simulink model "AB_Final_of_MPC_Bandwidth_Result_UnbalancedNew"  (R2022b)
settings: Solver=FixedStepDiscrete  StartTime=0.0  StopTime=Inf  FixedStep=100e-6  RelTol=1e-3  EnableMultiTasking=on
undefined symbols (not defined in the file): C28x, CPU1, CPU2, CurrentBypassValue, DiscIntNeverNeededParam, Down, GPTRIP1SEL, TZ1, Up
libraries: c2802xlib x20, simulink x17, dspstat3 x13, eeGeneralControl x10, c2837xDlib x5, c280xlib x5, PID_Lib x4, c2000lib x1, spsAlphaBetaZerotoabcLib x1
(part 2 of 10)

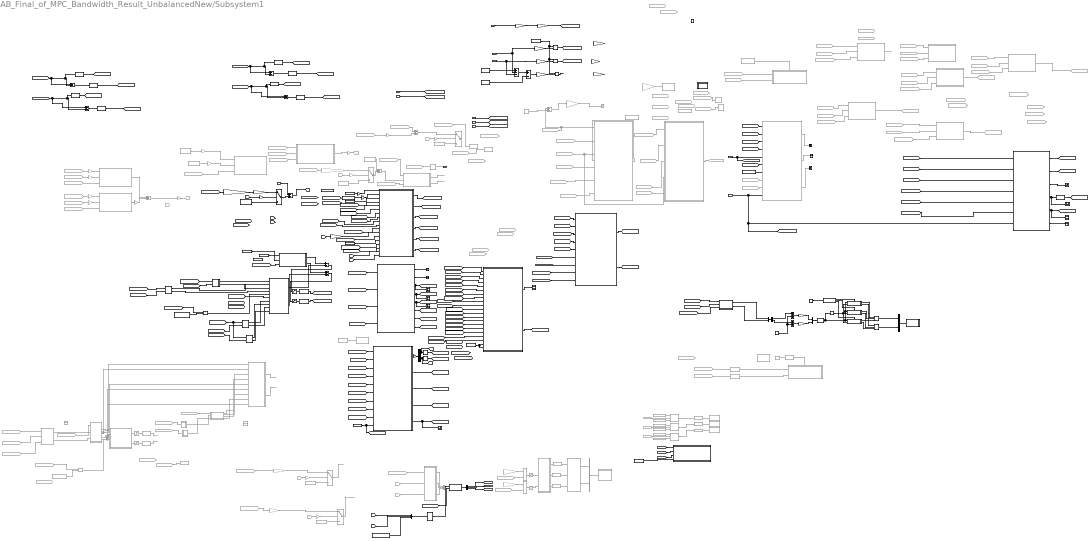
== system AB_Final_of_MPC_Bandwidth_Result_UnbalancedNew/Subsystem1 ==
  MPCC_f32GridCurrentA : Inport
  MPCC_f32GridCurrentB : Inport  Port=2
  PI_f32GridVoltageA : Inport  Port=3
  PI_f32GridVoltageB : Inport  Port=4
  PI_f32GridVoltageC : Inport  Port=5
  PI_f32DGridCurrentReference : Inport  Port=6
  PI_f32AngularFrequency : Inport  Port=7
  PI_f32ElectricalAngle : Inport  Port=8
  PI_f32DCLinkVoltage : Inport  Port=9
  PI_f32DCLinkVoltageref : Inport  Port=10
  MPCC_f32GridCurrentC : Inport  Port=11
  function : TriggerPort  TriggerType=function-call  VariantControl=(inherit)
  ABCtoAlphaBeta : Subsystem  Commented=on
  ABCtoD : Subsystem  Commented=on
  ABCtoD1Pos : Subsystem  Commented=on
  ABCtoD1Pos1 : Subsystem  Commented=on
  ABCtoD1Pos2 : Subsystem  Commented=on
  ABCtoD2 : Subsystem  Commented=on
  ABCtoD2Neg : Subsystem  Commented=on
  ABCtoD2Neg1 : Subsystem  Commented=on
  ABCtoD3 : Subsystem  Commented=on
  ABCtoDQO : Subsystem
  ABCtoQ : Subsystem  Commented=on
  ABCtoQPos1 : Subsystem  Commented=on
  Add1 : Sum  Inputs=+--
  Add{3,5,11,13..14} (5 alike) : Sum
  Add{4,6..7,12} (4 alike) : Sum  Commented=on
  Add{2,8..9,15..16} (5 alike) : Sum  Inputs=+-
  Alpha-Beta-Zero to abc : spsAlphaBetaZerotoabcLib/Alpha-Beta-Zero to abc
      settings: LibrarySourceBlock=|
      | sps_lib/Control/Alpha-Beta-Zero
      | to abc
  AlphaBetaDutiesCalculation : Subsystem
  AlphaBetaVoltageReferenceCalculation : Subsystem  Commented=on
  AlphaBetaVoltageReferenceCalculation1 : Subsystem
  "Angle_Identification " : Subsystem  Commented=on
  Bus Creator1 : BusCreator  Inputs=2
  Bus Selector2 : BusSelector  OutputSignals=signal1,signal2
  Cast To Boolean : DataTypeConversion  Commented=on  OutDataTypeStr=boolean  SaturateOnIntegerOverflow=off  RndMeth=Floor
  Cast To Single{,1..3,9..10,13..16,21} (11 alike) : DataTypeConversion  Commented=on  OutDataTypeStr=single  SaturateOnIntegerOverflow=off  RndMeth=Floor
  Cast To Single{6..8,11..12,17..20,22..23} (11 alike) : DataTypeConversion  OutDataTypeStr=single  SaturateOnIntegerOverflow=off  RndMeth=Floor
  CodeGeneration1 : Subsystem  TreatAsAtomicUnit=on
  Constant : Constant  Value=single(18.355e-3)
  Constant{1,10..11,14,48,50} (6 alike) : Constant  Value=single(0)
  Constant12 : Constant  Commented=on  Value=uint32(4999)
  Constant13 : Constant  Commented=on  Value=uint32(0)
  Constant{9,15,35,52,54} (5 alike) : Constant  Commented=on  Value=single(0)
  Constant16 : Constant  Commented=on  Value=uint32(4999)
  Constant17 : Constant  Commented=on  Value=uint32(0)
  Constant18 : Constant  Value=single(300)
  Constant19 : Constant  Value=single(9.5e-3)
  Constant2 : Constant  Value=single(0.005)
  Constant20 : Constant  Value=single(0.34)
  Constant21 : Constant  Value=single(18.5825e-3)
  Constant22 : Constant  Value=single(100e-6)
  Constant23 : Constant  Commented=on  Value=single(300)
  Constant26 : Constant  Value=single(1/10000)
  Constant3 : Constant  Value=10  OutDataTypeStr=single
  Constant36 : Constant  Commented=on
  Constant37 : Constant  Commented=on  Value=boolean(1)
  Constant4 : Constant  Commented=on  Value=single(1)  VectorParams1D=off  SampleTime=-1
  Constant45 : Constant  Commented=on  Value=single(-1)
  Constant46 : Constant  Value=boolean(0)
  Constant47 : Constant  Commented=on  Value=single(0.2)
  Constant5 : Constant  Commented=on  Value=10
  Constant51 : Constant  Value=single(1)
  Constant6 : Constant  Commented=on  Value=uint32(4999)
  Constant7 : Constant  Commented=on  Value=uint32(0)
  Constant8 : Constant  Commented=on  Value=single(80)
  Counter Limited1 : simulink/Sources/Counter Limited  uplimit=599  tsamp=-1
  DAC2 : c2837xDlib/DAC  Commented=on  channel=B  saturate=off
  Data Type Conversion18 : DataTypeConversion  Commented=on  OutDataTypeStr=uint32  SaturateOnIntegerOverflow=off  RndMeth=Floor
  Data Type Conversion19 : DataTypeConversion  Commented=on  OutDataTypeStr=uint32  SaturateOnIntegerOverflow=off  RndMeth=Floor
  Data Type Conversion5 : DataTypeConversion  Commented=on  OutDataTypeStr=uint32  SaturateOnIntegerOverflow=off  RndMeth=Floor
  Data1 : Subsystem  TreatAsAtomicUnit=on
  Data_Conditioning1 : Subsystem
  Decoupling_Loop : Subsystem  Commented=on
  Delay : Delay  DelayLength=1  InitialCondition=200
  Delay1 : Delay  DelayLength=1  InitialCondition=-200
  Demux : Demux  Outputs=2
  Demux1 : Demux  Outputs=3
  Digital Input : c280xlib/Digital Input  Commented=on  GPIO_Number=GPIO32~GPIO34  GPIO_Bit0=on  GPIO_Bit1=off  GPIO_Bit2=off  GPIO_Bit3=off  GPIO_Bit4=off  GPIO_Bit5=off  GPIO_Bit6=off  GPIO_Bit7=off  sampleTime=-1  dataType=boolean  GPIO_Bit0_Qualification=Sync to SYSCLKOUT  GPIO_Bit1_Qualification=Sync to SYSCLKOUT  GPIO_Bit2_Qualification=Sync to SYSCLKOUT  GPIO_Bit3_Qualification=Sync to SYSCLKOUT  GPIO_Bit4_Qualification=Sync to SYSCLKOUT  GPIO_Bit5_Qualification=Sync to SYSCLKOUT  GPIO_Bit6_Qualification=Sync to SYSCLKOUT  GPIO_Bit7_Qualification=Sync to SYSCLKOUT  Qualification_Period=-1
  Divide3 : Product  Commented=on  Inputs=*/  OutDataTypeStr=single  RndMeth=Zero  SaturateOnIntegerOverflow=on
  Divide5 : Product  Commented=on  Inputs=*/  OutDataTypeStr=single  RndMeth=Zero  SaturateOnIntegerOverflow=on
  End1 : Subsystem  TreatAsAtomicUnit=on
  From{1,31,96,128,168} (5 alike) : From  Commented=on  GotoTag=PI_f32DGridCurrentReference
  From10 : From  Commented=on  GotoTag=PWM1_Duty
  From{6,18,22,106,140,143,148,151,176} (9 alike) : From  Commented=on  GotoTag=PI_f32QGridCurrent
  From{11,19,137,173} (4 alike) : From  Commented=on  GotoTag=PI_f32QGridVoltage
  From123 : From  Commented=on  GotoTag=PI_f32GridVoltageA
  From{29,38,124,138,141,144,149,152,162,165,174} (11 alike) : From  Commented=on  GotoTag=MPCC_f32ElectricalAngle
  From{5,21,125,129,139,142,147,150,175} (9 alike) : From  Commented=on  GotoTag=PI_f32DGridCurrent
  From{20,24..25,126..127,189} (6 alike) : From  Commented=on  GotoTag=PI_f32DCLinkVoltage
  From13 : From  Commented=on  GotoTag=PI_f32DVoltage
  From{130,204,213,216,234} (5 alike) : From  Commented=on
  From131 : From  Commented=on  GotoTag=D
  From136 : From  Commented=on  GotoTag=PI_f32DGridVoltage
  From14 : From  Commented=on  GotoTag=PWM2_Duty
  From15 : From  Commented=on  GotoTag=PWM3_Duty
  From16 : From  Commented=on  GotoTag=PI_f32DCLinkVoltageref
  From163 : From  Commented=on  GotoTag=D1
  From164 : From  Commented=on  GotoTag=Q1
  From166 : From  Commented=on  GotoTag=D2
  From167 : From  Commented=on  GotoTag=Q2
  From169 : From  Commented=on  GotoTag=MPCC_f32DVoltageReference
  From170 : From  Commented=on  GotoTag=Q1
  From171 : From  Commented=on  GotoTag=D1
  From172 : From  Commented=on  GotoTag=PI_f32DGridVoltage
  From177 : From  Commented=on  GotoTag=D1
  From178 : From  Commented=on  GotoTag=Q1
  From181 : From  Commented=on  GotoTag=MPCC_f32ElectricalAngle_K_1
  From182 : From  Commented=on  GotoTag=PI_f32GridVoltageA
  From183 : From  Commented=on  GotoTag=PI_f32GridVoltageB
  From184 : From  Commented=on  GotoTag=MPCC_f32AngularFrequency
  From187 : From  Commented=on  GotoTag=PI_f32GridVoltageC
  From188 : From  Commented=on  GotoTag=FG
  From190 : From  Commented=on  GotoTag=FG
  From191 : From  Commented=on  GotoTag=IDD
  From192 : From  Commented=on  GotoTag=IQD
  From193 : From  Commented=on  GotoTag=MPCC_f32AngularFrequency
  From194 : From  Commented=on  GotoTag=MPCC_f32DConvVoltage
  From195 : From  Commented=on  GotoTag=MPCC_f32QConvVoltage
  From199 : From  Commented=on  GotoTag=D
  From200 : From  Commented=on  GotoTag=MPCC_f32QVoltageReference
  From206 : From  Commented=on  GotoTag=VQAC
  From212 : From
  From214 : From  Commented=on  GotoTag=MPCC_f32DVoltageReference
  From215 : From  Commented=on  GotoTag=VDAC
  From218 : From  Commented=on  GotoTag=MPCC_f32DVoltageReference
  From224 : From  Commented=on  GotoTag=VDD
  From225 : From  Commented=on  GotoTag=VQD
  From228 : From  Commented=on  GotoTag=VDD
  From229 : From  Commented=on  GotoTag=VQD
  From23 : From  Commented=on  GotoTag=PI_f32QVoltage
  From233 : From  Commented=on  GotoTag=IDD
  From236 : From  Commented=on  GotoTag=VDAC
  From237 : From  Commented=on  GotoTag=VQAC
  From238 : From  Commented=on  GotoTag=Q
  From26 : From  Commented=on  GotoTag=PI_f32GridCurrentA
  From27 : From  Commented=on  GotoTag=PI_f32GridCurrentB
  From28 : From  Commented=on  GotoTag=PI_f32GridCurrentC
  From3 : From  Commented=on  GotoTag=PI_f32QVoltage
  From30 : From  Commented=on  GotoTag=PI_f32DCLinkVoltageref
  From4 : From  Commented=on  GotoTag=PI_f32QGridCurrentReference
  From9 : From  Commented=on  GotoTag=PI_f32DGridVoltage
  From93 : From  Commented=on  GotoTag=MPCC_f32ElectricalAngle_K_1
  From97 : From  Commented=on  GotoTag=IQD
  Gain : Gain  Gain=single(-1)
  Gain1 : Gain  Gain=single(-1)
  Gain10 : Gain  Commented=on  Gain=single(4095/3.3)
  Gain11 : Gain  Gain=0.5
  Gain18 : Gain  Commented=on  Gain=single(2)
  Gain19 : Gain  Commented=on  Gain=single(2)
  Gain2 : Gain  Gain=single(6.25)
  Gain20 : Gain  Gain=single(5.85)
  Gain21 : Gain  Gain=single(1)
  Gain22 : Gain  Gain=single(1/30)
  Gain23 : Gain  Gain=-1
  Gain{24..29} (6 alike) : Gain  Commented=on
  Gain3 : Gain  Gain=single(5.94)
  Gain{31,39,50..51,53} (5 alike) : Gain  Commented=on  Gain=0
  Gain32 : Gain  Commented=on  Gain=-1
  Gain33 : Gain  Commented=on  Gain=-1
  Gain4 : Gain  Gain=single(5.94)
  Gain41 : Gain  Commented=on  Gain=single(-0.05)
  Gain46 : Gain  Gain=single(1)
  Gain47 : Gain  Gain=single(1)
  Gain49 : Gain  Gain=0
  Gain5 : Gain  Gain=single(-1)
  Gain52 : Gain  Commented=on  Gain=-5
  Gain54 : Gain  Commented=on  Gain=single(5)
  Gain55 : Gain  Commented=on  Gain=single(-5)
  Gain6 : Gain  Gain=1000  OutDataTypeStr=single
  Gain7 : Gain  Gain=1000  OutDataTypeStr=single
  Gain8 : Gain  Commented=on  Gain=single(4095/33)
  Gain9 : Gain  Gain=0.5
  Goto4 : Goto  Commented=on  GotoTag=PI_f32DVoltage
  Goto5 : Goto  Commented=on  GotoTag=PI_f32QVoltage
  Goto52 : Goto  Commented=on  GotoTag=D1
  Goto54 : Goto  Commented=on  GotoTag=Q1
  Goto55 : Goto  Commented=on  GotoTag=D2
  Goto56 : Goto  Commented=on  GotoTag=Q2
  Goto57 : Goto  Commented=on  GotoTag=ID2h
  Goto58 : Goto  Commented=on  GotoTag=IQ2h
  GridCurrentFirstPrediction : Subsystem
  GridCurrentSecondPrediction : Subsystem
  IPC Transmit : c2837xDlib/IPC Transmit  Commented=on  blkParamProc=F2837x  SelectDestination=C28x (CPU1/CPU2)  SelectChannel=0  EnableBlocking=off
  If1 : If  IfExpression=u1 == 0  ElseIfExpressions=u1 == 599
  LPF1 : DiscreteFilter  Commented=on  Numerator=[0 (2*pi*15*100e-6)]  Denominator=[1 (2*pi*15*100e-6-1)]  InitialStates=50/15/100e-6
  LPF3 : DiscreteFilter  Commented=on  Numerator=[0 (2*pi*15*100e-6)]  Denominator=[1 (2*pi*15*100e-6-1)]  InitialStates=50/15/100e-6
  MATLAB Function1 : MATLAB Function  Commented=on  TreatAsAtomicUnit=on
  MATLAB Function2 : MATLAB Function  Commented=on  TreatAsAtomicUnit=on
  MATLAB Function3 : MATLAB Function  TreatAsAtomicUnit=on
  Merge2 : Merge  Inputs=3
  Merge3 : Merge  Inputs=3
  ModulatorTimes : Subsystem
  Moving Average1 : dspstat3/Moving Average  Commented=on  Method=Exponential weighting  ForgettingFactorPort=off  SpecifyWindowLength=on  WindowLength=4  OverlapLength=3  AllowArbitraryInputLength=off  ForgettingFactor=0.99  SimulateUsing=Code generation
  Moving Average2 : dspstat3/Moving Average  Commented=on  Method=Exponential weighting  ForgettingFactorPort=off  SpecifyWindowLength=on  WindowLength=4  OverlapLength=3  AllowArbitraryInputLength=off  ForgettingFactor=0.99  SimulateUsing=Code generation
  Mux1 : Mux  Inputs=2
  Mux3 : Mux  Commented=on  Inputs=2
  Mux4 : Mux  Commented=on  Inputs=3
  Mux5 : Mux  Inputs=2
  Mux6 : Mux  Inputs=3
  PI_DGridCurrent : Subsystem  Commented=on
  PI_QGridCurrent : Subsystem  Commented=on
  PSCE : Subsystem  Commented=on
  PSCE1 : Subsystem  Commented=on
  Product{,1..2,4} (4 alike) : Product
  Product3 : Product  Commented=on
  SOGI 1st6 : Subsystem
  SOGI 1st7 : Subsystem
  SOGI 1st8 : Subsystem
  SOGI 1st9 : Subsystem
  SVM : Subsystem
  SVPWM : Subsystem  Commented=on
  Saturation : Saturate  Commented=on  UpperLimit=single(2/sqrt(3))  LowerLimit=single(-2/sqrt(3))
  Saturation Dynamic1 : simulink/Discontinuities/Saturation Dynamic  Commented=on  OutMin=[]  OutMax=[]  OutDataTypeStr=Inherit: Same as second input  OutDataType=fixdt(1, 16)  OutScaling=2^-10  DoSatur=off
  Saturation Dynamic2 : simulink/Discontinuities/Saturation Dynamic  Commented=on  OutMin=[]  OutMax=[]  OutDataTypeStr=Inherit: Same as second input  OutDataType=fixdt(1, 16)  OutScaling=2^-10  DoSatur=off
  Saturation Dynamic3 : simulink/Discontinuities/Saturation Dynamic  Commented=on  OutMin=[]  OutMax=[]  OutDataTypeStr=Inherit: Same as second input  OutDataType=fixdt(1, 16)  OutScaling=2^-10  DoSatur=off
  Saturation3 : Saturate  Commented=on  UpperLimit=single(2/sqrt(3))  LowerLimit=single(-2/sqrt(3))
  Saturation4 : Saturate  Commented=on  UpperLimit=7  LowerLimit=-7
  Saturation5 : Saturate  Commented=on  UpperLimit=7  LowerLimit=-7
  Saturation6 : Saturate  UpperLimit=7  LowerLimit=-7
  Saturation7 : Saturate  UpperLimit=7  LowerLimit=-7
  Scope{,1..6} (7 alike) : Scope
  Signal Copy1 : SignalConversion  Commented=on  OverrideOpt=off
  Start1 : Subsystem  TreatAsAtomicUnit=on
  Subsystem : Subsystem
  Subsystem1 : Subsystem  Commented=on
  Subsystem2 : Subsystem  Commented=on
  Subsystem3 : Subsystem  Commented=on
  Subsystem4 : Subsystem  Commented=on
  Subsystem6 : Subsystem
  Switch : Switch  Criteria=u2 ~= 0  SaturateOnIntegerOverflow=off  InputSameDT=off
  Switch1 : Switch  Commented=on  Criteria=u2 ~= 0  SaturateOnIntegerOverflow=off  InputSameDT=off
  Switch4 : Switch  Commented=on  Criteria=u2 ~= 0  OutDataTypeStr=Inherit: Inherit via back propagation  SaturateOnIntegerOverflow=off  InputSameDT=off
  Switch5 : Switch  Commented=on  Criteria=u2 ~= 0  OutDataTypeStr=Inherit: Inherit via back propagation  SaturateOnIntegerOverflow=off  InputSameDT=off
  Switch6 : Switch  Commented=on  Criteria=u2 ~= 0  OutDataTypeStr=Inherit: Inherit via back propagation  SaturateOnIntegerOverflow=off  InputSameDT=off
  System Outputs : Subsystem  mask(System Outputs){ShowInLibBrowser=0}
      mask prompts: ShowInLibBrowser "Simulink:masks:CustCodeMaskParam1_MP"
      settings: CopyFcn=cccopyfcn(gcb)  OpenFcn=ccopenfcn('System Outputs Function')
      mask Help: eval('feval(''rtwprivate'',''rtwhelpview'',''rtw_sys_outputs_block'')');
      mask Display: disp('System\nOutputs');
  Terminator : Terminator  Commented=on
  Terminator{3..7,10..11} (7 alike) : Terminator
  VoltageReferenceCalculation : Subsystem
  Width1 : Width  OutDataTypeMode=All ports same datatype  DataType=uint16
  dq_abc : Subsystem  Commented=on
  dq_abc1 : Subsystem  Commented=on
  ePWM5 : c2802xlib/ePWM  Commented=on  PwmType=C2000_Type4  useModule=ePWM1  ePWMxLINKTBPRD=Not Linked  periodUnits=Clock cycles  timerSource=Specify via dialog  timerPeriod_clk=5000  timerPeriod_sec=0.0001  tbshadow=Counter equals to zero  countingMode=Up-Down  phaseActiveEnable=Disable  phaseDirection=Count down after sync  phaseActive=0  synchronizationEnable=off  dcaevt1Sync=off  dcbevt1Sync=off  synchronizationOption=Disable  dcbevt1SyncOut=off  dcaevt1SyncOut=off  cmpdSyncOut=off  cmpcSyncOut=off  cmpbSyncOut=off  zeroSyncOut=off  swfSyncOut=off  perSynchronizationOption=Counter equals to period (CTR=PRD)  clockPrescale=1  HSclockPrescale=1  enswap=off  ePWMxAStatus=on  ePWMxAactionLogic1=Do nothing  ePWMxAactionLogic2=Do nothing  ePWMxAactionLogic3=Clear  ePWMxAactionLogic4=Set  ePWMxAactionLogic5=Do nothing  ePWMxAactionLogic6=Do nothing  ePWMxACSFenable=off  ePWMxACSFvalue=Forcing disable  ePWMxASFreload=Zero  ePWMxBStatus=off  ePWMxBactionLogic1=Set  ePWMxBactionLogic2=Clear  ePWMxBactionLogic3=Do nothing  ePWMxBactionLogic4=Do nothing  ePWMxBactionLogic5=Clear  ePWMxBactionLogic6=Set  ePWMxBCSFenable=off  ePWMxBCSFvalue=Forcing disable  ePWMxBSFreload=Zero  ePWNxBOutWay=off  ePWMxLINKCMPA=Not Linked  CMPAUnits=Clock cycles  CMPASource=Input port  CMPAValue_per=50  CMPAValue_clk=0  enCMPAshadow=Counter equals to zero (CTR=Zero)  ePWMxLINKCMPB=Not Linked  CMPBUnits=Clock cycles  CMPBSource=Specify via dialog  CMPBValue_per=50  CMPBValue_clk=0  enCMPBshadow=Counter equals to zero (CTR=Zero)  ePWMxLINKCMPC=Not Linked  CMPCUnits=Clock cycles  CMPCSource=Specify via dialog  CMPCValue_per=50  CMPCValue_clk=0  enCMPCshadow=Counter equals to zero (CTR=Zero)  ePWMxLINKCMPD=Not Linked  CMPDUnits=Clock cycles  CMPDSource=Specify via dialog  CMPDValue_per=50  CMPDValue_clk=32000  enCMPDshadow=Counter equals to zero (CTR=Zero)  enableDBePWMxA=on  enableDBePWMxB=on  enhalfcycle=off  DBpolarity=Active high complementary (AHC)  DBedgeDelay=Positive  DBSource_ePWMxA=ePWMxA  DBSource_ePWMxB=ePWMxA  DBPeriodUnits=Clock cycles  DBperiodSource=Specify via dialog  REDperiod=250  FEDperiod=250  REDperiod_sec=0  FEDperiod_sec=0  LoadModeDBRED=Immediate without using shadow  LoadModeDBFED=Immediate without using shadow  adcstartModuleA=on  adcrequestEventA=First event  adcstartEventA=Digital Compare Module A Event 1 start of conversion (DCAEVT1.soc)  adcstartEventA_type2=Counter equals to period (CTR=PRD)  adcstartModuleB=off  adcrequestEventB=First event  adcstartEventB=Counter equals to zero (CTR=Zero)  adcstartEventB_type2=Counter equals to zero (CTR=Zero)  intEn=off  intPrd=First event  intSel=Counter equals to zero (CTR=Zero)  intSel_type2=Counter equals to zero (CTR=Zero)  hrpe=off  enHRPWM=off  HRPWM_LoadMode=Counter equals to period (CTR=PRD)  HRPWM_CTLMode=Duty or Period control mode  HRPWM_EDGMode=Both edge  hrpeb=off  enHRPWMB=off  HRPWM_LoadModeB=Counter equals to zero (CTR=ZERO)  HRPWM_CTLModeB=Duty or Period control mode  HRPWM_EDGModeB=Both edge  enHRDBRED=off  enHRDBFED=off  enSFO=on  enautoconv=on  chopperEnable=off  chopperFrequency=1  chopperFirstwidth=1  chopperDuty=12.5%  tripZonesource=Specify via dialog  tzselOSHT1=off  tzselOSHT2=off  tzselOSHT3=off  tzselOSHDCAEV1=off  tzselOSHDCBEV1=off  tzselCBC1=off  tzselCBC2=off  tzselCBC3=off  tzselCBCDCAEV2=off  tzselCBCDCBEV2=off  tzselOSHT4=off  tzselOSHT5=off  tzselOSHT6=off  tzselCBC4=off  tzselCBC5=off  tzselCBC6=off  enTzOstIntr=off  enTzCbcIntr=off  enTzDCAEVT1Intr=off  enTzDCAEVT2Intr=off  enTzDCBEVT1Intr=off  enTzDCBEVT2Intr=off  ePWMxAforced=No action  ePWMxBforced=No action  DCAEVT1forced=No action  DCBEVT1forced=No action  DCAEVT2forced=No action  DCBEVT2forced=No action  dcah=Trip Zone 1 input (TZ1)  dcal=Trip Zone 2 input (TZ2)  dcbh=Trip Zone 1 input (TZ1)  dcbl=Trip Zone 2 input (TZ2)  dcah_type2=GPTRIP1SEL/(TZ1)  dcal_type2=GPTRIP1SEL/(TZ1)  dcbh_type2=GPTRIP1SEL/(TZ1)  dcbl_type2=GPTRIP1SEL/(TZ1)  gendcaevt1=Event disabled  gendcaevt2=Event disabled  gendcbevt1=Event disabled  gendcbevt2=Event disabled  dcaevt1src=DCAEVT1 with sync  dcaevt2src=DCAEVT2 with sync  dcbevt1src=DCBEVT1 with sync  dcbevt2src=DCBEVT2 with sync  pulsesel=Counter equals to zero (CTR=Zero)  blankinv=off  blankoffset=0  blankwidth=0  evsrcsel=Filtered version of DCAEVT1 (DCAEVT1FILT)  encape=off
  ePWM6 : c2802xlib/ePWM  Commented=on  PwmType=C2000_Type4  useModule=ePWM2  ePWMxLINKTBPRD=Not Linked  periodUnits=Clock cycles  timerSource=Specify via dialog  timerPeriod_clk=5000  timerPeriod_sec=0.0001  tbshadow=Counter equals to zero  countingMode=Up-Down  phaseActiveEnable=Disable  phaseDirection=Count down after sync  phaseActive=0  synchronizationEnable=off  dcaevt1Sync=off  dcbevt1Sync=off  synchronizationOption=Disable  dcbevt1SyncOut=off  dcaevt1SyncOut=off  cmpdSyncOut=off  cmpcSyncOut=off  cmpbSyncOut=off  zeroSyncOut=off  swfSyncOut=off  perSynchronizationOption=Counter equals to period (CTR=PRD)  clockPrescale=1  HSclockPrescale=1  enswap=off  ePWMxAStatus=on  ePWMxAactionLogic1=Do nothing  ePWMxAactionLogic2=Do nothing  ePWMxAactionLogic3=Clear  ePWMxAactionLogic4=Set  ePWMxAactionLogic5=Do nothing  ePWMxAactionLogic6=Do nothing  ePWMxACSFenable=off  ePWMxACSFvalue=Forcing disable  ePWMxASFreload=Zero  ePWMxBStatus=off  ePWMxBactionLogic1=Set  ePWMxBactionLogic2=Clear  ePWMxBactionLogic3=Do nothing  ePWMxBactionLogic4=Do nothing  ePWMxBactionLogic5=Clear  ePWMxBactionLogic6=Set  ePWMxBCSFenable=off  ePWMxBCSFvalue=Forcing disable  ePWMxBSFreload=Zero  ePWNxBOutWay=off  ePWMxLINKCMPA=Not Linked  CMPAUnits=Clock cycles  CMPASource=Input port  CMPAValue_per=50  CMPAValue_clk=0  enCMPAshadow=Counter equals to zero (CTR=Zero)  ePWMxLINKCMPB=Not Linked  CMPBUnits=Clock cycles  CMPBSource=Specify via dialog  CMPBValue_per=50  CMPBValue_clk=0  enCMPBshadow=Counter equals to zero (CTR=Zero)  ePWMxLINKCMPC=Not Linked  CMPCUnits=Clock cycles  CMPCSource=Specify via dialog  CMPCValue_per=50  CMPCValue_clk=0  enCMPCshadow=Counter equals to zero (CTR=Zero)  ePWMxLINKCMPD=Not Linked  CMPDUnits=Clock cycles  CMPDSource=Specify via dialog  CMPDValue_per=50  CMPDValue_clk=32000  enCMPDshadow=Counter equals to zero (CTR=Zero)  enableDBePWMxA=on  enableDBePWMxB=on  enhalfcycle=off  DBpolarity=Active high complementary (AHC)  DBedgeDelay=Positive  DBSource_ePWMxA=ePWMxA  DBSource_ePWMxB=ePWMxA  DBPeriodUnits=Clock cycles  DBperiodSource=Specify via dialog  REDperiod=250  FEDperiod=250  REDperiod_sec=0  FEDperiod_sec=0  LoadModeDBRED=Immediate without using shadow  LoadModeDBFED=Immediate without using shadow  adcstartModuleA=off  adcrequestEventA=First event  adcstartEventA=Digital Compare Module A Event 1 start of conversion (DCAEVT1.soc)  adcstartEventA_type2=Counter equals to zero (CTR=Zero)  adcstartModuleB=off  adcrequestEventB=First event  adcstartEventB=Counter equals to zero (CTR=Zero)  adcstartEventB_type2=Counter equals to zero (CTR=Zero)  intEn=off  intPrd=First event  intSel=Counter equals to zero (CTR=Zero)  intSel_type2=Counter equals to zero (CTR=Zero)  hrpe=off  enHRPWM=off  HRPWM_LoadMode=Counter equals to period (CTR=PRD)  HRPWM_CTLMode=Duty or Period control mode  HRPWM_EDGMode=Both edge  hrpeb=off  enHRPWMB=off  HRPWM_LoadModeB=Counter equals to zero (CTR=ZERO)  HRPWM_CTLModeB=Duty or Period control mode  HRPWM_EDGModeB=Both edge  enHRDBRED=off  enHRDBFED=off  enSFO=on  enautoconv=on  chopperEnable=off  chopperFrequency=1  chopperFirstwidth=1  chopperDuty=12.5%  tripZonesource=Specify via dialog  tzselOSHT1=off  tzselOSHT2=off  tzselOSHT3=off  tzselOSHDCAEV1=off  tzselOSHDCBEV1=off  tzselCBC1=off  tzselCBC2=off  tzselCBC3=off  tzselCBCDCAEV2=off  tzselCBCDCBEV2=off  tzselOSHT4=off  tzselOSHT5=off  tzselOSHT6=off  tzselCBC4=off  tzselCBC5=off  tzselCBC6=off  enTzOstIntr=off  enTzCbcIntr=off  enTzDCAEVT1Intr=off  enTzDCAEVT2Intr=off  enTzDCBEVT1Intr=off  enTzDCBEVT2Intr=off  ePWMxAforced=No action  ePWMxBforced=No action  DCAEVT1forced=No action  DCBEVT1forced=No action  DCAEVT2forced=No action  DCBEVT2forced=No action  dcah=Trip Zone 1 input (TZ1)  dcal=Trip Zone 2 input (TZ2)  dcbh=Trip Zone 1 input (TZ1)  dcbl=Trip Zone 2 input (TZ2)  dcah_type2=GPTRIP1SEL/(TZ1)  dcal_type2=GPTRIP1SEL/(TZ1)  dcbh_type2=GPTRIP1SEL/(TZ1)  dcbl_type2=GPTRIP1SEL/(TZ1)  gendcaevt1=Event disabled  gendcaevt2=Event disabled  gendcbevt1=Event disabled  gendcbevt2=Event disabled  dcaevt1src=DCAEVT1 with sync  dcaevt2src=DCAEVT2 with sync  dcbevt1src=DCBEVT1 with sync  dcbevt2src=DCBEVT2 with sync  pulsesel=Counter equals to zero (CTR=Zero)  blankinv=off  blankoffset=0  blankwidth=0  evsrcsel=Filtered version of DCAEVT1 (DCAEVT1FILT)  encape=off
  ePWM7 : c2802xlib/ePWM  Commented=on  PwmType=C2000_Type4  useModule=ePWM3  ePWMxLINKTBPRD=Not Linked  periodUnits=Clock cycles  timerSource=Specify via dialog  timerPeriod_clk=5000  timerPeriod_sec=0.0001  tbshadow=Counter equals to zero  countingMode=Up-Down  phaseActiveEnable=Disable  phaseDirection=Count down after sync  phaseActive=0  synchronizationEnable=off  dcaevt1Sync=off  dcbevt1Sync=off  synchronizationOption=Disable  dcbevt1SyncOut=off  dcaevt1SyncOut=off  cmpdSyncOut=off  cmpcSyncOut=off  cmpbSyncOut=off  zeroSyncOut=off  swfSyncOut=off  perSynchronizationOption=Counter equals to period (CTR=PRD)  clockPrescale=1  HSclockPrescale=1  enswap=off  ePWMxAStatus=on  ePWMxAactionLogic1=Do nothing  ePWMxAactionLogic2=Do nothing  ePWMxAactionLogic3=Clear  ePWMxAactionLogic4=Set  ePWMxAactionLogic5=Do nothing  ePWMxAactionLogic6=Do nothing  ePWMxACSFenable=off  ePWMxACSFvalue=Forcing disable  ePWMxASFreload=Zero  ePWMxBStatus=off  ePWMxBactionLogic1=Set  ePWMxBactionLogic2=Clear  ePWMxBactionLogic3=Do nothing  ePWMxBactionLogic4=Do nothing  ePWMxBactionLogic5=Clear  ePWMxBactionLogic6=Set  ePWMxBCSFenable=off  ePWMxBCSFvalue=Forcing disable  ePWMxBSFreload=Zero  ePWNxBOutWay=off  ePWMxLINKCMPA=Not Linked  CMPAUnits=Clock cycles  CMPASource=Input port  CMPAValue_per=50  CMPAValue_clk=0  enCMPAshadow=Counter equals to zero (CTR=Zero)  ePWMxLINKCMPB=Not Linked  CMPBUnits=Clock cycles  CMPBSource=Specify via dialog  CMPBValue_per=50  CMPBValue_clk=0  enCMPBshadow=Counter equals to zero (CTR=Zero)  ePWMxLINKCMPC=Not Linked  CMPCUnits=Clock cycles  CMPCSource=Specify via dialog  CMPCValue_per=50  CMPCValue_clk=0  enCMPCshadow=Counter equals to zero (CTR=Zero)  ePWMxLINKCMPD=Not Linked  CMPDUnits=Clock cycles  CMPDSource=Specify via dialog  CMPDValue_per=50  CMPDValue_clk=32000  enCMPDshadow=Counter equals to zero (CTR=Zero)  enableDBePWMxA=on  enableDBePWMxB=on  enhalfcycle=off  DBpolarity=Active high complementary (AHC)  DBedgeDelay=Positive  DBSource_ePWMxA=ePWMxA  DBSource_ePWMxB=ePWMxA  DBPeriodUnits=Clock cycles  DBperiodSource=Specify via dialog  REDperiod=250  FEDperiod=250  REDperiod_sec=0  FEDperiod_sec=0  LoadModeDBRED=Immediate without using shadow  LoadModeDBFED=Immediate without using shadow  adcstartModuleA=off  adcrequestEventA=First event  adcstartEventA=Digital Compare Module A Event 1 start of conversion (DCAEVT1.soc)  adcstartEventA_type2=Counter equals to zero (CTR=Zero)  adcstartModuleB=off  adcrequestEventB=First event  adcstartEventB=Counter equals to zero (CTR=Zero)  adcstartEventB_type2=Counter equals to zero (CTR=Zero)  intEn=off  intPrd=First event  intSel=Counter equals to zero (CTR=Zero)  intSel_type2=Counter equals to zero (CTR=Zero)  hrpe=off  enHRPWM=off  HRPWM_LoadMode=Counter equals to period (CTR=PRD)  HRPWM_CTLMode=Duty or Period control mode  HRPWM_EDGMode=Both edge  hrpeb=off  enHRPWMB=off  HRPWM_LoadModeB=Counter equals to zero (CTR=ZERO)  HRPWM_CTLModeB=Duty or Period control mode  HRPWM_EDGModeB=Both edge  enHRDBRED=off  enHRDBFED=off  enSFO=on  enautoconv=on  chopperEnable=off  chopperFrequency=1  chopperFirstwidth=1  chopperDuty=12.5%  tripZonesource=Specify via dialog  tzselOSHT1=off  tzselOSHT2=off  tzselOSHT3=off  tzselOSHDCAEV1=off  tzselOSHDCBEV1=off  tzselCBC1=off  tzselCBC2=off  tzselCBC3=off  tzselCBCDCAEV2=off  tzselCBCDCBEV2=off  tzselOSHT4=off  tzselOSHT5=off  tzselOSHT6=off  tzselCBC4=off  tzselCBC5=off  tzselCBC6=off  enTzOstIntr=off  enTzCbcIntr=off  enTzDCAEVT1Intr=off  enTzDCAEVT2Intr=off  enTzDCBEVT1Intr=off  enTzDCBEVT2Intr=off  ePWMxAforced=No action  ePWMxBforced=No action  DCAEVT1forced=No action  DCBEVT1forced=No action  DCAEVT2forced=No action  DCBEVT2forced=No action  dcah=Trip Zone 1 input (TZ1)  dcal=Trip Zone 2 input (TZ2)  dcbh=Trip Zone 1 input (TZ1)  dcbl=Trip Zone 2 input (TZ2)  dcah_type2=GPTRIP1SEL/(TZ1)  dcal_type2=GPTRIP1SEL/(TZ1)  dcbh_type2=GPTRIP1SEL/(TZ1)  dcbl_type2=GPTRIP1SEL/(TZ1)  gendcaevt1=Event disabled  gendcaevt2=Event disabled  gendcbevt1=Event disabled  gendcbevt2=Event disabled  dcaevt1src=DCAEVT1 with sync  dcaevt2src=DCAEVT2 with sync  dcbevt1src=DCBEVT1 with sync  dcbevt2src=DCBEVT2 with sync  pulsesel=Counter equals to zero (CTR=Zero)  blankinv=off  blankoffset=0  blankwidth=0  evsrcsel=Filtered version of DCAEVT1 (DCAEVT1FILT)  encape=off
  nominal : Constant  Value=single(0.7)
  underload : Constant  Value=single(0.1)
  Out1 : Outport
  wires:
  Add1/1 -> Add2/1
  Constant2/1 -> Add2/2
  Add2/1 -> Gain4/1
  MPCC_f32GridCurrentA/1 -> Gain2/1, Add1/2
  MPCC_f32GridCurrentB/1 -> Add1/3, Gain3/1
  Constant1/1 -> Add1/1
  [PI_f32QGridVoltage] -> Decoupling_Loop/4(PI_f32QGridVoltage)
  From3/1 -> Decoupling_Loop/9(PI_f32QVoltage)
  From4/1 -> PI_QGridCurrent/1(PI_f32QGridCurrentReference)
  [PI_f32QGridCurrent] -> Decoupling_Loop/2(PI_f32QGridCurrent)
  From6/1 -> PI_QGridCurrent/2(PI_f32QGridCurrent)
  [PI_f32DGridVoltage] -> Decoupling_Loop/3(PI_f32DGridVoltage)
  Constant/1 -> Decoupling_Loop/7(PI_f32LGrid)
  [PI_f32DCLinkVoltage] -> Decoupling_Loop/6(PI_f32DCLinkVoltage)
  [PI_f32DGridCurrent] -> Decoupling_Loop/1(PI_f32DGridCurrent)
  PI_QGridCurrent/1(PI_f32QVoltage) -> Goto5/1
  PI_f32AngularFrequency/1 -> [MPCC_f32AngularFrequency], Decoupling_Loop/5(PI_f32AngularFrequency)
  PI_DGridCurrent/1(PI_f32DVoltage) -> Goto4/1
  From13/1 -> Decoupling_Loop/8(PI_f32DVoltage)
  [PI_f32GridCurrentA] -> ABCtoDQO/1(PI_f32GridCurrentA)
  ABCtoDQO/6(PI_f32OGridVoltage) -> Terminator6/1
  [PI_f32GridVoltageB] -> ABCtoDQO/5(PI_f32GridVoltageB)
  ABCtoDQO/1(PI_f32DGridCurrent) -> [PI_f32DGridCurrent]
  [PI_f32GridVoltageC] -> ABCtoDQO/6(PI_f32GridVoltageC)
  ABCtoDQO/5(PI_f32QGridVoltage) -> Scope4/1, [PI_f32QGridVoltage]
  [PI_f32GridCurrentB] -> ABCtoDQO/2(PI_f32GridCurrentB)
  [PI_f32GridCurrentC] -> ABCtoDQO/3(PI_f32GridCurrentC)
  ABCtoDQO/3(PI_f32OGridCurrent) -> Terminator7/1
  ABCtoDQO/2(PI_f32QGridCurrent) -> [PI_f32QGridCurrent]
  ABCtoDQO/4(PI_f32DGridVoltage) -> Scope3/1, Cast To Single6/1
  PI_f32GridVoltageC/1 -> [PI_f32GridVoltageC]
  PI_f32GridVoltageB/1 -> [PI_f32GridVoltageB]
  PI_f32GridVoltageA/1 -> [PI_f32GridVoltageA]
  PI_f32ElectricalAngle/1 -> [MPCC_f32ElectricalAngle], ABCtoDQO/7(PI_f32ElectricalAngle), Decoupling_Loop/10(PI_f32ElectricalAngle)
  From5/1 -> Add4/1, PI_DGridCurrent/1(PI_f32DGridCurrent)
  PI_f32DCLinkVoltage/1 -> [PI_f32DCLinkVoltage]
  From9/1 -> PI_QGridCurrent/4(PI_f32DGridVoltage), PI_DGridCurrent/3(PI_f32DGridVoltage)
  From11/1 -> PI_QGridCurrent/3(PI_f32QGridVoltage)
  From19/1 -> PI_DGridCurrent/4(PI_f32QGridVoltage)
  [PI_f32GridVoltageA] -> ABCtoDQO/4(PI_f32GridVoltageA)
  Gain8/1 -> Terminator/1
  Add4/1 -> Gain8/1
  Constant5/1 -> Add4/2
  Gain10/1 -> DAC2/1
  From20/1 -> PI_DGridCurrent/5(PI_f32DCLinkVoltage)
  From23/1 -> PI_DGridCurrent/6(PI_f32QVoltage)
  From24/1 -> PI_QGridCurrent/5(PI_f32DCLinkVoltage)
  From1/1 -> PI_DGridCurrent/2(PI_f32DGridCurrentReference)
  From25/1 -> Moving Average1/1
  From31/1 -> Moving Average2/1
  VoltageReferenceCalculation/5(MPCC_f32Predictionterm_B) -> [MPCC_f32Predictionterm_B]
  [PI_f32QGridCurrentReference] -> VoltageReferenceCalculation/13(MPCC_f32QGridCurrentReference)
  Gain22/1 -> VoltageReferenceCalculation/12(MPCC_f32HarmonicDGridCurrentReference)
  VoltageReferenceCalculation/4(MPCC_f32Predictionterm_A) -> [MPCC_f32Predictionterm_A]
  Constant22/1 -> VoltageReferenceCalculation/3(MPCC_f32SamplingPeriod)
  [MPCC_f32AngularFrequency] -> VoltageReferenceCalculation/4(MPCC_f32AngularFrequency)
  VoltageReferenceCalculation/3(MPCC_f32ElectricalAngle_K_1) -> [MPCC_f32ElectricalAngle_K_1]
  Constant10/1 -> VoltageReferenceCalculation/14(MPCC_f32HarmonicQGridCurrentReference)
  VoltageReferenceCalculation/6(MPCC_f32Predictionterm_C) -> [MPCC_f32Predictionterm_C]
  Constant20/1 -> Gain9/1
  [MPCC_f32ElectricalAngle] -> VoltageReferenceCalculation/15(MPCC_f32ElectricalAngle)
  [PI_f32DGridCurrentReference] -> VoltageReferenceCalculation/11(MPCC_f32DGridCurrentReference)
  GridCurrentFirstPrediction/1(MPCC_f32DGridCurrent_K_1) -> [MPCC_f32DGridCurrent_K_1]
  [MPCC_f32Predictionterm_A] -> GridCurrentFirstPrediction/1(MPCC_f32Predictionterm_A)
  [MPCC_f32Predictionterm_C] -> GridCurrentFirstPrediction/3(MPCC_f32Predictionterm_C)
  [PI_f32DGridCurrent] -> GridCurrentFirstPrediction/4(MPCC_f32DGridCurrent)
  [MPCC_f32Predictionterm_B] -> GridCurrentFirstPrediction/2(MPCC_f32Predictionterm_B)
  [PI_f32QGridCurrent] -> GridCurrentFirstPrediction/5(MPCC_f32QGridCurrent)
  GridCurrentFirstPrediction/2(MPCC_f32QGridCurrent_K_1) -> [MPCC_f32QGridCurrent_K_1]
  [PI_f32DCLinkVoltage] -> AlphaBetaDutiesCalculation/4(MPCC_f32DCLinkVoltage)
  [MPCC_f32ElectricalAngle_K_1] -> AlphaBetaDutiesCalculation/3(MPCC_f32ElectricalAngle_K_1)
  AlphaBetaDutiesCalculation/3(MPCC_f32Duty_Sector1) -> Scope1/1, [MPCC_f32Duty_Sector1]
  AlphaBetaDutiesCalculation/4(MPCC_f32Duty_Sector2) -> Scope2/1, [MPCC_f32Duty_Sector2]
  [MPCC_f32DVoltageReference] -> AlphaBetaDutiesCalculation/1(MPCC_f32DVoltageReference)
  [MPCC_f32QVoltageReference] -> AlphaBetaDutiesCalculation/2(MPCC_f32QVoltageReference)
  AlphaBetaDutiesCalculation/8(MPCC_f32Duty_Sector6) -> [MPCC_f32Duty_Sector6]
  AlphaBetaDutiesCalculation/6(MPCC_f32Duty_Sector4) -> [MPCC_f32Duty_Sector4]
  AlphaBetaDutiesCalculation/2(MPCC_f32BetaVoltageReference) -> Terminator11/1
  AlphaBetaDutiesCalculation/5(MPCC_f32Duty_Sector3) -> Scope5/1, [MPCC_f32Duty_Sector3]
  AlphaBetaDutiesCalculation/7(MPCC_f32Duty_Sector5) -> [MPCC_f32Duty_Sector5]
  AlphaBetaDutiesCalculation/1(MPCC_f32AlphaVoltageReference) -> Terminator10/1
  [MPCC_f32Predictionterm_B] -> GridCurrentSecondPrediction/3(MPCC_f32Predictionterm_B)
  [PI_f32DCLinkVoltage] -> GridCurrentSecondPrediction/11(MPCC_f32DCLinkVoltage)
  [MPCC_f32Duty_Sector2] -> GridCurrentSecondPrediction/13(MPCC_f32Duty_Sector2)
  [MPCC_f32Duty_Sector6] -> GridCurrentSecondPrediction/17(MPCC_f32Duty_Sector6)
  [MPCC_f32QGridCurrent_K_1] -> GridCurrentSecondPrediction/6(MPCC_f32QGridCurrent_K_1)
  GridCurrentSecondPrediction/1(MPCC_f32MinCostFunction) -> Scope6/1
  [PI_f32QGridCurrentReference] -> GridCurrentSecondPrediction/8(MPCC_f32QGridCurrentReference)
  [MPCC_f32Duty_Sector4] -> GridCurrentSecondPrediction/15(MPCC_f32Duty_Sector4)
  [MPCC_f32Predictionterm_C] -> GridCurrentSecondPrediction/4(MPCC_f32Predictionterm_C)
  [MPCC_f32ElectricalAngle_K_1] -> GridCurrentSecondPrediction/1(MPCC_f32ElectricalAngle_K_1)
  [MPCC_f32Duty_Sector3] -> GridCurrentSecondPrediction/14(MPCC_f32Duty_Sector3)
  [PI_f32DGridCurrentReference] -> GridCurrentSecondPrediction/7(MPCC_f32DGridCurrentReference)
  [MPCC_f32Duty_Sector5] -> GridCurrentSecondPrediction/16(MPCC_f32Duty_Sector5)
  [MPCC_f32Predictionterm_A] -> GridCurrentSecondPrediction/2(MPCC_f32Predictionterm_A)
  [MPCC_f32Duty_Sector1] -> GridCurrentSecondPrediction/12(MPCC_f32Duty_Sector1)
  [MPCC_f32DGridCurrent_K_1] -> GridCurrentSecondPrediction/5(MPCC_f32DGridCurrent_K_1)
  Delay/1 -> [MPCC_f32DConvVoltage]
  ModulatorTimes/4(MPCC_f32Time0) -> [MPCC_f32Time0]
  [MPCC_f32Duty_Sector6] -> ModulatorTimes/8(MPCC_f32Duty_Sector6)
  ModulatorTimes/1(MPCC_f32DQConvVoltage) -> Gain23/1
  Constant26/1 -> [MPCC_f32SwitchingPeriod], ModulatorTimes/10(MPCC_f32SwitchingPeriod)
  ModulatorTimes/2(MPCC_f32Time1) -> [MPCC_f32Time1]
  [MPCC_f32Duty_Sector1] -> ModulatorTimes/3(MPCC_f32Duty_Sector1)
  [MPCC_f32ElectricalAngle_K_1] -> ModulatorTimes/1(MPCC_f32ElectricalAngle_K_1)
  Delay1/1 -> [MPCC_f32QConvVoltage]
  ModulatorTimes/5(MPCC_u8ModulationSector) -> Scope/1, [MPCC_u8ModulationSector]
  [MPCC_f32MinSector] -> ModulatorTimes/9(MPCC_f32MinSector)
  [MPCC_f32Duty_Sector2] -> ModulatorTimes/4(MPCC_f32Duty_Sector2)
  [MPCC_f32Duty_Sector5] -> ModulatorTimes/7(MPCC_f32Duty_Sector5)
  [MPCC_f32Duty_Sector4] -> ModulatorTimes/6(MPCC_f32Duty_Sector4)
  [PI_f32DCLinkVoltage] -> ModulatorTimes/2(MPCC_f32DCLinkVoltage)
  ModulatorTimes/3(MPCC_f32Time2) -> [MPCC_f32Time2]
  [MPCC_f32Duty_Sector3] -> ModulatorTimes/5(MPCC_f32Duty_Sector3)
  Decoupling_Loop/2(PI_f32MBVoltageRef) -> Terminator4/1
  Decoupling_Loop/1(PI_f32MAVoltageRef) -> Terminator3/1
  Decoupling_Loop/3(PI_f32MCVoltageRef) -> Terminator5/1
  Demux/1 -> [D], Delay/1
  Cast To Single6/1 -> [PI_f32DGridVoltage]
  GridCurrentSecondPrediction/2(MPCC_f32MinSector) -> [MPCC_f32MinSector]
  Data Type Conversion5/1 -> ePWM5/1
  Constant17/1 -> Saturation Dynamic2/3
  From14/1 -> Saturation Dynamic2/2
  Saturation Dynamic3/1 -> Data Type Conversion19/1
  From10/1 -> Saturation Dynamic1/2
  Constant7/1 -> Saturation Dynamic1/3
  Saturation Dynamic2/1 -> Data Type Conversion18/1
  Saturation Dynamic1/1 -> Data Type Conversion5/1
  From15/1 -> Saturation Dynamic3/2
  Constant12/1 -> Saturation Dynamic3/1
  Constant16/1 -> Saturation Dynamic2/1
  Constant6/1 -> Saturation Dynamic1/1
  Constant13/1 -> Saturation Dynamic3/3
  Data Type Conversion19/1 -> ePWM7/1
  Data Type Conversion18/1 -> ePWM6/1
  [PI_f32DCLinkVoltage] -> VoltageReferenceCalculation/16(MPCC_f32DCLinkVoltage)
  PI_f32DCLinkVoltageref/1 -> [PI_f32DCLinkVoltageref]
  Cast To Boolean/1 -> Subsystem1/Enable
  Cast To Single9/1 -> Subsystem1/1(In1)
  Cast To Single10/1 -> Subsystem1/2(In2)
  [PWM3_Duty] -> Subsystem/3(PWM3)
  [PWM2_Duty] -> Subsystem/2(PWM2)
  [PWM1_Duty] -> Subsystem/1(PWM1)
  From124/1 -> Cast To Single10/1
  From123/1 -> Cast To Single9/1
  Constant36/1 -> Cast To Boolean/1
  Constant37/1 -> Subsystem2/Enable
  From128/1 -> Subsystem2/1(In1)
  From129/1 -> Subsystem2/2(In2)
  From125/1 -> Signal Copy1/1
  Signal Copy1/1 -> Out1/1
  Cast To Single1/1 -> "Angle_Identification "/1(A)
  dq_abc/1(Ia) -> Cast To Single1/1
  ? -> dq_abc/1(theta)
  "Angle_Identification "/1(V_alpha) -> Mux3/1
  Cast To Single3/1 -> "Angle_Identification "/3(C)
  dq_abc/2(Ib) -> Cast To Single2/1
  "Angle_Identification "/2(V_beta) -> Mux3/2
  Cast To Single2/1 -> "Angle_Identification "/2(B)
  Divide3/1 -> Saturation/1
  Mux3/1 -> SVPWM/1(Valpha_beta)
  dq_abc/3(Ic) -> Cast To Single3/1
  Gain18/1 -> Divide3/1
  From126/1 -> Divide3/2
  From127/1 -> Divide5/2
  Gain19/1 -> Divide5/1
  Demux/2 -> [Q], Delay1/1
  Constant46/1 -> Subsystem/4(Trip)
  Gain2/1 -> Product/2  "Iau"
  Product/1 -> [PI_f32GridCurrentA]
  Gain3/1 -> Product1/2  "Ibu"
  Product1/1 -> [PI_f32GridCurrentB]
  Gain4/1 -> Product2/2  "Icu"
  Product2/1 -> ?
  Constant51/1 -> Product2/1, Product1/1, Product/1
  Divide5/1 -> Saturation3/1
  Saturation3/1 -> dq_abc/3(vq)
  Saturation/1 -> dq_abc/2(vd)
  MPCC_f32GridCurrentC/1 -> Gain20/1
  Gain20/1 -> Gain21/1  "Iau"
  Gain21/1 -> [PI_f32GridCurrentC]  "Iau"
  From38/1 -> ABCtoQ/3(MPCC_f32ElectricalAngle)
  Constant47/1 -> Gain33/1
  From29/1 -> ABCtoD/3(MPCC_f32ElectricalAngle)
  Constant52/1 -> Switch1/3
  ABCtoQ/1(MPCC_f32HarmonicQGridCurrent) -> Gain28/1
  Switch/1 -> Add5/2
  PI_f32DGridCurrentReference/1 -> Add5/1
  Switch1/1 -> Add6/2
  Constant4/1 -> Add6/1
  Constant45/1 -> Gain32/1
  From141/1 -> ABCtoD2Neg/3(MPCC_f32ElectricalAngle)
  From140/1 -> ABCtoD2Neg/2(MPCC_f32QGridCurrent)
  From139/1 -> ABCtoD2Neg/1(MPCC_f32DGridCurrent)
  From175/1 -> ABCtoD1Pos/1(MPCC_f32DGridCurrent)
  From138/1 -> ABCtoD1Pos/3(MPCC_f32ElectricalAngle)
  From176/1 -> ABCtoD1Pos/2(MPCC_f32QGridCurrent)
  ABCtoD1Pos/1(MPCC_f32HarmonicDGridCurrent) -> Goto52/1
  From142/1 -> ABCtoQPos1/1(MPCC_f32DGridCurrent)
  From144/1 -> ABCtoQPos1/3(MPCC_f32ElectricalAngle)
  From143/1 -> ABCtoQPos1/2(MPCC_f32QGridCurrent)
  ABCtoQPos1/1(MPCC_f32HarmonicQGridCurrent) -> Goto54/1
  From147/1 -> ABCtoD1Pos1/1(MPCC_f32DGridCurrent)
  From149/1 -> ABCtoD1Pos1/3(MPCC_f32ElectricalAngle)
  From148/1 -> ABCtoD1Pos1/2(MPCC_f32QGridCurrent)
  From150/1 -> ABCtoD2Neg1/1(MPCC_f32DGridCurrent)
  From152/1 -> ABCtoD2Neg1/3(MPCC_f32ElectricalAngle)
  From151/1 -> ABCtoD2Neg1/2(MPCC_f32QGridCurrent)
  ABCtoD1Pos1/1(MPCC_f32HarmonicDGridCurrent) -> Goto55/1
  ABCtoD2Neg1/1(MPCC_f32HarmonicDGridCurrent) -> Goto56/1
  From162/1 -> ABCtoD2/3(MPCC_f32ElectricalAngle)
  From163/1 -> Gain24/1
  From164/1 -> Gain25/1
  From166/1 -> Gain26/1
  From165/1 -> ABCtoD3/3(MPCC_f32ElectricalAngle)
  From167/1 -> Gain27/1
  Gain24/1 -> ABCtoD2/1(MPCC_f32DGridCurrent)
  Gain25/1 -> ABCtoD2/2(MPCC_f32QGridCurrent)
  Gain26/1 -> ABCtoD3/1(MPCC_f32DGridCurrent)
  Gain27/1 -> ABCtoD3/2(MPCC_f32QGridCurrent)
  ABCtoD2/1(MPCC_f32HarmonicDGridCurrent) -> Add7/1
  ABCtoD3/1(MPCC_f32HarmonicDGridCurrent) -> Gain31/1
  Add7/1 -> Gain29/1
  Gain31/1 -> Add7/2
  Gain32/1 -> ABCtoD/1(MPCC_f32DGridCurrent)
  Gain33/1 -> ABCtoD/2(MPCC_f32QGridCurrent)
  From172/1 -> ABCtoD1Pos2/1(MPCC_f32DGridCurrent)
  From174/1 -> ABCtoD1Pos2/3(MPCC_f32ElectricalAngle)
  From173/1 -> ABCtoD1Pos2/2(MPCC_f32QGridCurrent)
  ABCtoD1Pos2/1(MPCC_f32HarmonicDGridCurrent) -> ?
  From177/1 -> ABCtoQ/1(MPCC_f32DGridCurrent)
  From178/1 -> ABCtoQ/2(MPCC_f32QGridCurrent)
  Gain29/1 -> Goto57/1
  Gain28/1 -> Goto58/1
  Constant50/1 -> Switch/3
  [VDAC] -> VoltageReferenceCalculation/17(MPCC_f32HarmonicDGridVoltage)
  [VQAC] -> VoltageReferenceCalculation/18(MPCC_f32HarmonicQGridVoltage)
  Add8/1 -> Cast To Single11/1
  [PI_f32QGridVoltage] -> Cast To Single17/1, Add9/2, Add9/1
  Add9/1 -> Cast To Single12/1
  From212/1 -> Gain49/1
  Cast To Single12/1 -> [VQAC]
  Gain46/1 -> Switch/1
  Gain41/1 -> Switch1/1
  Cast To Single11/1 -> [VDAC]
  [PI_f32DGridVoltage] -> Cast To Single18/1, Add8/2, Add8/1
  [VDAC] -> Gain47/1
  Gain47/1 -> Gain46/1
  From206/1 -> Gain41/1
  From213/1 -> Gain50/1
  Gain49/1 -> Switch/2
  Gain50/1 -> Switch1/2
  Constant35/1 -> Switch4/3
  Gain51/1 -> Switch4/2
  From216/1 -> Gain51/1
  From215/1 -> Gain52/1
  From214/1 -> Add12/1
  Add12/1 -> Switch4/1
  From96/1 -> Cast To Single16/1
  Gain52/1 -> Add12/2
  Cast To Single17/1 -> [VQD]
  Cast To Single18/1 -> [VDD]
  [PI_f32QGridVoltage] -> GridCurrentFirstPrediction/7(MPCC_f32QGridVoltage)
  [PI_f32DGridVoltage] -> GridCurrentFirstPrediction/6(MPCC_f32DGridVoltage)
  [PI_f32DGridVoltage] -> GridCurrentSecondPrediction/9(MPCC_f32DGridVoltage)
  [PI_f32QGridVoltage] -> GridCurrentSecondPrediction/10(MPCC_f32QGridVoltage)
  From233/1 -> Cast To Single14/1
  Gain39/1 -> Switch5/2
  Constant15/1 -> Switch5/3
  Gain54/1 -> Switch5/1
  From236/1 -> Gain54/1
  From130/1 -> Gain39/1
  Switch5/1 -> ?
  Gain53/1 -> Switch6/2
  Constant54/1 -> Switch6/3
  Gain55/1 -> Switch6/1
  Switch6/1 -> ?
  From237/1 -> Gain55/1
  From234/1 -> Gain53/1
  [VDAC] -> Gain22/1
  [VDD] -> VoltageReferenceCalculation/9(MPCC_f32DGridVoltage)
  [VQD] -> VoltageReferenceCalculation/10(MPCC_f32QGridVoltage)
  [PI_f32DGridCurrent] -> Cast To Single20/1, Add15/2, Add15/1
  Cast To Single20/1 -> [IDD]
  [PI_f32QGridCurrent] -> Cast To Single19/1, Add16/2, Add16/1
  Cast To Single19/1 -> [IQD]
  Add15/1 -> Cast To Single7/1
  Cast To Single8/1 -> [IQAC]
  Add16/1 -> Cast To Single8/1
  Cast To Single7/1 -> [IDAC]
  [IDAC] -> VoltageReferenceCalculation/7(MPCC_f32HarmonicDGridCurrent)
  [IQAC] -> VoltageReferenceCalculation/8(MPCC_f32HarmonicQGridCurrent)
  Gain23/1 -> Demux/1
  From131/1 -> dq_abc1/2(vd)
  From238/1 -> dq_abc1/3(vq)
  From93/1 -> dq_abc1/1(theta)
  dq_abc1/2(Ib) -> Mux4/2
  dq_abc1/3(Ic) -> Mux4/3
  dq_abc1/1(Ia) -> Mux4/1
  [PI_f32DCLinkVoltage] -> SVM/2(Vdc)
  SVM/1(Dabc) -> Demux1/1
  Demux1/1 -> [PWM1_Duty]
  Demux1/2 -> [PWM2_Duty]
  Demux1/3 -> [PWM3_Duty]
  Constant48/1 -> Mux6/3
  Mux6/1 -> Alpha-Beta-Zero to abc/1
  [D] -> Mux6/1
  [Q] -> Mux6/2
  Alpha-Beta-Zero to abc/1 -> SVM/1(Vabc)
  Add6/1 -> AlphaBetaVoltageReferenceCalculation/2(MPCC_f32QVoltageReference)
  From181/1 -> AlphaBetaVoltageReferenceCalculation/3(MPCC_f32ElectricalAngle_K_1)
  ABCtoAlphaBeta/1(alpha) -> PSCE/2(alpha)
  From184/1 -> PSCE/1(w)
  ABCtoAlphaBeta/2(Vαβ) -> PSCE/3(beta)
  From182/1 -> ABCtoAlphaBeta/1(In1)
  From183/1 -> ABCtoAlphaBeta/2(In2)
  From187/1 -> ABCtoAlphaBeta/3(In3)
  PSCE/3(Ealpha) -> MATLAB Function1/1(e_alpha), MATLAB Function2/1(Ealpha)
  PSCE/5(Ealpha_) -> MATLAB Function2/2(Ealpha_), MATLAB Function1/2(e_alpha_prime)
  PSCE/7(Ebeta) -> MATLAB Function1/5(e_beta), MATLAB Function2/3(Ebeta)
  PSCE/8(Ebeta_) -> MATLAB Function2/4(Ebeta_), MATLAB Function1/6(e_beta_prime)
  Add5/1 -> [FG]
  Product3/1 -> MATLAB Function2/5(Pref), MATLAB Function1/9(Pref)
  MATLAB Function2/1(alpha) -> Saturation4/1
  MATLAB Function2/2(beta) -> Saturation5/1
  From190/1 -> AlphaBetaVoltageReferenceCalculation/1(MPCC_f32DVoltageReference)
  VoltageReferenceCalculation/1(MPCC_f32DVoltageReference) -> [MPCC_f32DVoltageReference]
  VoltageReferenceCalculation/2(MPCC_f32QVoltageReference) -> [MPCC_f32QVoltageReference]
  Cast To Single21/1 -> ?
  Cast To Single/1 -> ?
  From192/1 -> Cast To Single15/1
  Saturation4/1 -> Cast To Single/1
  Saturation5/1 -> Cast To Single21/1
  From188/1 -> Product3/1
  Constant23/1 -> Product3/2
  PSCE1/4(betan) -> MATLAB Function1/8(v_beta_prime)
  From193/1 -> PSCE1/1(w)
  PSCE1/2(betap) -> MATLAB Function1/7(v_beta)
  PSCE1/3(alphan) -> MATLAB Function1/4(v_alpha_prime)
  PSCE1/1(alphap) -> MATLAB Function1/3(v_alpha)
  From194/1 -> Subsystem3/1(In1)
  From195/1 -> Subsystem4/1(In1)
  Subsystem3/1(alpha) -> PSCE1/2(alpha)
  Subsystem4/1(beta) -> PSCE1/3(beta)
  MATLAB Function1/1(alpha) -> ?
  MATLAB Function1/2(beta) -> ?
  [MPCC_f32DConvVoltage] -> GridCurrentFirstPrediction/8(MPCC_f32DConvVoltage)
  [MPCC_f32QConvVoltage] -> GridCurrentFirstPrediction/9(MPCC_f32QConvVoltage)
  AlphaBetaVoltageReferenceCalculation/1(MPCC_f32AlphaVoltageReference) -> ?
  AlphaBetaVoltageReferenceCalculation/2(MPCC_f32BetaVoltageReference) -> ?
  Constant11/1 -> GridCurrentSecondPrediction/21(MPCC_f32QGridCurrent1), GridCurrentSecondPrediction/20(MPCC_f32DGridCurrent1)
  Saturation7/1 -> Cast To Single23/1
  Saturation6/1 -> Cast To Single22/1
  Cast To Single23/1 -> [PI_f32QGridCurrentReference]
  Cast To Single22/1 -> [PI_f32DGridCurrentReference]
  [FG] -> Product4/1
  Constant18/1 -> Product4/2
  Product4/1 -> MATLAB Function3/5(Pref)
  [MPCC_f32AngularFrequency] -> MATLAB Function3/6(omega)
  [MPCC_f32AngularFrequency] -> SOGI 1st7/1(w), SOGI 1st6/1(w)
  [IDD] -> SOGI 1st6/2(Vαβ)
  [IQD] -> SOGI 1st7/2(Vαβ)
  Constant19/1 -> Gain11/1
  Cast To Single13/1 -> IPC Transmit/1
  Constant14/1 -> AlphaBetaVoltageReferenceCalculation1/1(MPCC_f32DVoltageReference)
  [MPCC_f32ElectricalAngle_K_1] -> AlphaBetaVoltageReferenceCalculation1/3(MPCC_f32ElectricalAngle_K_1)
  AlphaBetaVoltageReferenceCalculation1/1(MPCC_f32AlphaVoltageReference) -> Add11/1
  AlphaBetaVoltageReferenceCalculation1/2(MPCC_f32BetaVoltageReference) -> Add13/1
  MATLAB Function3/1(alpha) -> Add11/2
  Add11/1 -> Saturation6/1
  MATLAB Function3/2(beta) -> Add13/2
  Add13/1 -> Saturation7/1
  [IDD] -> VoltageReferenceCalculation/5(MPCC_f32DGridCurrent)
  [IQD] -> VoltageReferenceCalculation/6(MPCC_f32QGridCurrent)
  [IDD] -> GridCurrentSecondPrediction/18(MPCC_f32DGridCurrent)
  [IQD] -> GridCurrentSecondPrediction/19(MPCC_f32QGridCurrent)
  [MPCC_f32AngularFrequency] -> SOGI 1st8/1(w)
  SOGI 1st9/1(v) -> MATLAB Function3/1(ea)
  SOGI 1st9/2(qv) -> MATLAB Function3/3(ea_p)
  [MPCC_f32AngularFrequency] -> SOGI 1st9/1(w)
  [VDD] -> SOGI 1st9/2(Vαβ)
  [VQD] -> SOGI 1st8/2(Vαβ)
  SOGI 1st8/2(qv) -> MATLAB Function3/4(eb_p)
  SOGI 1st8/1(v) -> MATLAB Function3/2(eb)
  SOGI 1st6/1(v) -> MATLAB Function3/7(ia)
  SOGI 1st6/2(qv) -> MATLAB Function3/9(ia1)
  SOGI 1st7/2(qv) -> MATLAB Function3/10(ib1)
  SOGI 1st7/1(v) -> MATLAB Function3/8(ib)
  [MPCC_f32ElectricalAngle] -> Subsystem6/3(theta)
  Bus Selector2/2 -> Add14/1  "<signal2>"
  Mux1/1 -> CodeGeneration1/1(Input)
  Subsystem6/2(Iq) -> Bus Creator1/2
  Start1/1(Data_out) -> Merge2/1
  [PI_f32DGridCurrent] -> Subsystem6/1(In1)
  If1/1 -> Start1/Action
  Add3/1 -> Gain7/1
  Mux5/1 -> Data_Conditioning1/1(In1)
  Gain6/1 -> Mux5/2
  Subsystem6/1(Id) -> Bus Creator1/1
  If1/3 -> Data1/Action
  If1/2 -> End1/Action
  Gain7/1 -> Mux5/1
  Data1/2(Iteration) -> Merge3/3
  Bus Selector2/1 -> Add3/1  "<signal1>"
  Add14/1 -> Gain6/1
  Bus Creator1/1 -> Bus Selector2/1
  Constant3/1 -> Add3/2, Add14/2
  Data_Conditioning1/1(Out1) -> Width1/1, Start1/1(Data), End1/1(Data), Data1/1(Data)
  Data1/1(Data_out) -> Merge2/3
  Merge3/1 -> Mux1/2  "SCI_Tx_Iteration"
  [PI_f32QGridCurrent] -> Subsystem6/2(In2)
  Counter Limited1/1 -> If1/1
  Merge2/1 -> Mux1/1  "SCI_Tx_Data"
  Width1/1 -> Data1/2(Data_width), Start1/2(Data_width), End1/2(Data_width)
  End1/1(Data_out) -> Merge2/2
  End1/2(Iteration) -> Merge3/2
  Start1/2(Iteration) -> Merge3/1
  nominal/1 -> AlphaBetaVoltageReferenceCalculation1/2(MPCC_f32QVoltageReference)
  Gain9/1 -> VoltageReferenceCalculation/1(MPCC_f32RGrid)
  Gain11/1 -> VoltageReferenceCalculation/2(MPCC_f32LGrid)

== system AB_Final_of_MPC_Bandwidth_Result_UnbalancedNew/Subsystem2 ==
  function : TriggerPort  TriggerType=function-call  VariantControl=(inherit)
  Constant : Constant  Value=boolean(1)
  Digital Output : c2837xDlib/Digital Output  GPIO_Number=GPIO8~GPIO15  GPIO_Bit0=off  GPIO_BIT0_Toggle=off  GPIO_Bit1=off  GPIO_BIT1_Toggle=off  GPIO_Bit2=off  GPIO_BIT2_Toggle=off  GPIO_Bit3=off  GPIO_BIT3_Toggle=off  GPIO_Bit4=off  GPIO_BIT4_Toggle=off  GPIO_Bit5=off  GPIO_BIT5_Toggle=off  GPIO_Bit6=on  GPIO_BIT6_Toggle=off  GPIO_Bit7=off  GPIO_BIT7_Toggle=off
  wires:
  Constant/1 -> Digital Output/1
